simulink model "engine_test"  (R2020a)
settings: Solver=ode23tb  StartTime=0.0  StopTime=20  MaxStep=tsample
libraries: nesl_utility x5, fl_lib x2, Liebherr_Engine_D934_lib x1
settings Model: SimulationMode=accelerator  Creator=dbagn  LastModifiedBy=dbagn
settings DataIOCC: SaveTime=off  ReturnWorkspaceOutputs=off
settings SFSimCC: SimCustomHeaderCode="#include \"sfbctrl.h\""  SimUserSources=src/sfbctrl.c  SimUserIncludeDirs=include

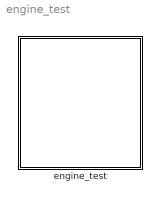
== system engine_test ==
  engine_test : Subsystem

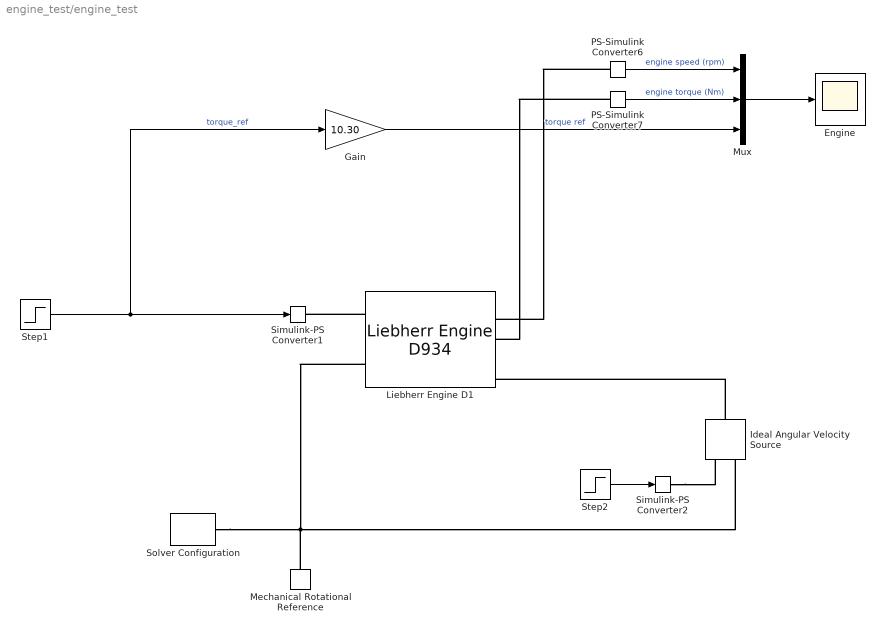
== system engine_test/engine_test ==
  Engine : Scope
  Gain : Gain  Gain=10.30
  Ideal Angular Velocity Source : fl_lib/Mechanical/Mechanical Sources/Ideal Angular Velocity Source
  Liebherr Engine D1 : Liebherr_Engine_D934_lib/Liebherr Engine D934  dynamic_response=simscape.enum.onoff.on  cshaft_inertia=1 kg*m^2  initial_speed=1
      settings: InternalSimscapePortConfiguration="{\"Bottom\":[],\"Left\":[{\"id\":\"tS\",\"label\":\"tS\",\"type\":\"input\"},{\"id\":\"C\",\"label\":\"C\",\"type\":\"foundation.mechanical.rotational.rotational\"}],\"Right\":[{\"id\":\"Po\",\"label\":\"PE\",\"type\":\"output\"},{\"id\":\"wE\",\"label\":\"wE\",\"type\":\"output\"},{\"id\":\"tE\",\"label\":\"tE\",\"type\":\"output\"},{\"id\":\"eE\",\"label\":\"eE\",\"type\":\"output\"},{\"id\":\"D\",\"label\":\"D\",\"type\":\"foundation.mechanical.rotational.rotational\"}],\"Top\":[]}"
  Mechanical Rotational Reference : fl_lib/Mechanical/Rotational Elements/Mechanical Rotational Reference
  Mux : Mux  Inputs=3
  PS-Simulink Converter6 : nesl_utility/PS-Simulink Converter  PhysicalDomain=network_engine_domain  SubClassName=ps_output  LeftPortType=input  RightPortType=output  PseudoPeriodic=off  Frequencies=[]  Unit=inherit  AffineConversion=off
  PS-Simulink Converter7 : nesl_utility/PS-Simulink Converter  PhysicalDomain=network_engine_domain  SubClassName=ps_output  LeftPortType=input  RightPortType=output  PseudoPeriodic=off  Frequencies=[]  Unit=inherit  AffineConversion=off
  Simulink-PS Converter1 : nesl_utility/Simulink-PS Converter  PhysicalDomain=network_engine_domain  SubClassName=ps_input  LeftPortType=input  RightPortType=output  PseudoPeriodic=off  Frequencies=[]  NoiseDistribution=none  NoiseParameters=[]  Unit=1  AffineConversion=off  FilteringAndDerivatives=provide  SimscapeFilterOrder=2  InputFilterTimeConstant=0.1  UdotUserProvided=0
  Simulink-PS Converter2 : nesl_utility/Simulink-PS Converter  PhysicalDomain=network_engine_domain  SubClassName=ps_input  LeftPortType=input  RightPortType=output  PseudoPeriodic=off  Frequencies=[]  NoiseDistribution=none  NoiseParameters=[]  Unit=rpm  AffineConversion=off  FilteringAndDerivatives=filter  SimscapeFilterOrder=2  InputFilterTimeConstant=0.1  UdotUserProvided=0
  Solver Configuration : nesl_utility/Solver Configuration  PhysicalDomain=network_engine_domain  SubClassName=solver  LeftPortType=input  RightPortType=generic  Tones=[]  Harmonics=[]  SimulateNoise=off  Profile=off  UseLocalSampling=off  EnableSwitchedLinearOptims=on  FrequencyDomain=off  UseCCode=off  RelTol=0.001  AbsTol=1e-06  MinStep=1e-09  ToWorkspace=off  RevertToSquareIcSolve=off  NumHomotopyIterations=100  PhasorMode=off  PhasorModeNumHarmonics=1  DoDC=off  ResidualTolerance=1e-09  UseLocalSolver=on  LocalSolverChoice=NE_BACKWARD_EULER_ADVANCER  LocalSolverSampleTime=tsample  DoFixedCost=on  MaxNonlinIter=3  MaxModeIter=2  LinearAlgebra=auto  EquationFormulation=NE_TIME_EF  DelaysMemoryBudget=1024  AutomaticFiltering=on  FilteringTimeConstant=tsample  PartitionStorageMethod=AS_NEEDED  PartitionMemoryBudget=1024  PartitionMethod=ROBUST
  Step1 : Step  Time=10  After=100  SampleTime=0
  Step2 : Step  Before=800  After=1900  SampleTime=0
  wires:
  Step1/1 -> Simulink-PS Converter1/1, Gain/1  "torque_ref"
  PS-Simulink Converter6/1 -> Mux/1  "engine speed (rpm)"
  PS-Simulink Converter7/1 -> Mux/2  "engine torque (Nm)"
  Mux/1 -> Engine/1
  Step2/1 -> Simulink-PS Converter2/1
  Gain/1 -> Mux/3  "torque ref"
  connections:
  Ideal Angular Velocity Source/LConn1 -- Liebherr Engine D1/RConn5
  PS-Simulink Converter6/LConn1 -- Liebherr Engine D1/RConn2
  Liebherr Engine D1/LConn1 -- Simulink-PS Converter1/RConn1
  Mechanical Rotational Reference/LConn1 -- Liebherr Engine D1/LConn2 -- Ideal Angular Velocity Source/RConn2 -- Solver Configuration/RConn1
  PS-Simulink Converter7/LConn1 -- Liebherr Engine D1/RConn3
  Simulink-PS Converter2/RConn1 -- Ideal Angular Velocity Source/RConn1
